simulink model "SpringMassSystemContrlledByPID"  (R2016b)
settings: Solver=ode45  StartTime=0.0  StopTime=50  MaxStep=0.05  RelTol=1e-3
libraries: simulink x1
settings Model: Creator=shyam  LastModifiedBy=shyam

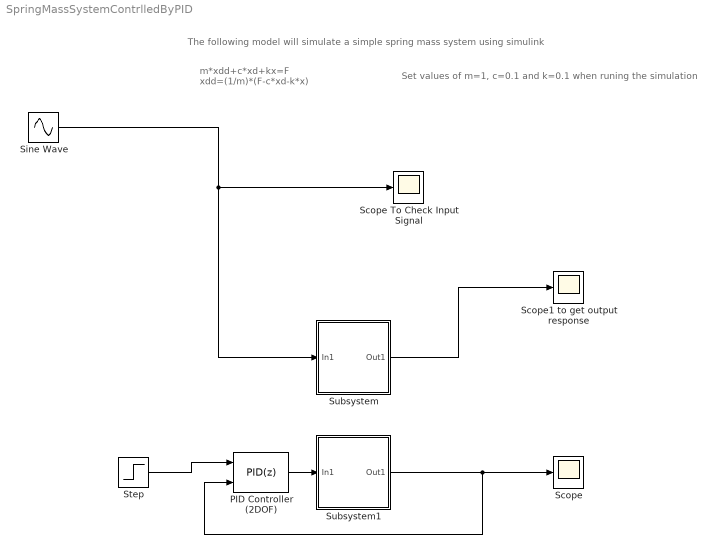
== system SpringMassSystemContrlledByPID ==
  note: Set values of m=1, c=0.1 and k=0.1 when runing the simulation
  note: The following model will simulate a simple spring mass system using simulink
  note: m*xdd+c*xd+kx=F
      | xdd=(1/m)*(F-c*xd-k*x)
  PID Controller (2DOF) : simulink/Continuous/PID Controller (2DOF)  Controller=PID  TimeDomain=Discrete-time  SampleTime=0.01  IntegratorMethod=Forward Euler  FilterMethod=Forward Euler  Form=Parallel  UseFilter=on  ControllerParametersSource=internal  P=3.93514485654865  I=0.388930047898937  D=7.6285518493241  N=88.4850232977662  b=0.926545410813894  c=0.00568917134188472  InitialConditionSource=internal  InitialConditionForIntegrator=0  InitialConditionForFilter=0  ExternalReset=none  LimitOutput=off  UpperSaturationLimit=inf  LowerSaturationLimit=-inf  LinearizeAsGain=on  AntiWindupMode=none  Kb=1  TrackingMode=off  Kt=1  PParamMin=[]  PParamMax=[]  IParamMin=[]  IParamMax=[]  DParamMin=[]  DParamMax=[]  NParamMin=[]  NParamMax=[]  bParamMin=[]  bParamMax=[]  cParamMin=[]  cParamMax=[]  KbParamMin=[]  KbParamMax=[]  KtParamMin=[]  KtParamMax=[]  POutMin=[]  POutMax=[]  IOutMin=[]  IOutMax=[]  DOutMin=[]  DOutMax=[]  NOutMin=[]  NOutMax=[]  bOutMin=[]  bOutMax=[]  cOutMin=[]  cOutMax=[]  KbOutMin=[]  KbOutMax=[]  KtOutMin=[]  KtOutMax=[]  IntegratorOutMin=[]  IntegratorOutMax=[]  FilterOutMin=[]  FilterOutMax=[]  SumOutMin=[]  SumOutMax=[]  Sum1OutMin=[]  Sum1OutMax=[]  Sum2OutMin=[]  Sum2OutMax=[]  Sum3OutMin=[]  Sum3OutMax=[]  SumI1OutMin=[]  SumI1OutMax=[]  SumI2OutMin=[]  SumI2OutMax=[]  SumI3OutMin=[]  SumI3OutMax=[]  SumDOutMin=[]  SumDOutMax=[]  SaturationOutMin=[]  SaturationOutMax=[]  IntegratorContinuousStateAttributes=''  IntegratorStateMustResolveToSignalObject=off  IntegratorRTWStateStorageClass=Auto  FilterContinuousStateAttributes=''  FilterStateMustResolveToSignalObject=off  FilterRTWStateStorageClass=Auto  DifferentiatorICPrevScaledInput=0  DifferentiatorOutMin=[]  DifferentiatorOutMax=[]
  Scope : Scope
  "Scope To Check Input Signal " : Scope
  "Scope1 to get output response " : Scope
  Sine Wave : Sin  Amplitude=2  SampleTime=0
  Step : Step  SampleTime=0
  Subsystem : Subsystem  mask{m=6, k=0.5, c=3}
      mask prompts: m "Mass"; k "Spring"; c "Damper"
  Subsystem1 : Subsystem  mask{m=6, k=0.5, c=0.1}
      mask prompts: m "Mass"; k "Spring"; c "Damper"
  wires:
  Sine Wave/1 -> Subsystem/1(In1), "Scope To Check Input Signal "/1
  Subsystem/1(Out1) -> "Scope1 to get output response "/1
  Step/1 -> PID Controller (2DOF)/1
  Subsystem1/1(Out1) -> PID Controller (2DOF)/2, Scope/1
  PID Controller (2DOF)/1 -> Subsystem1/1(In1)

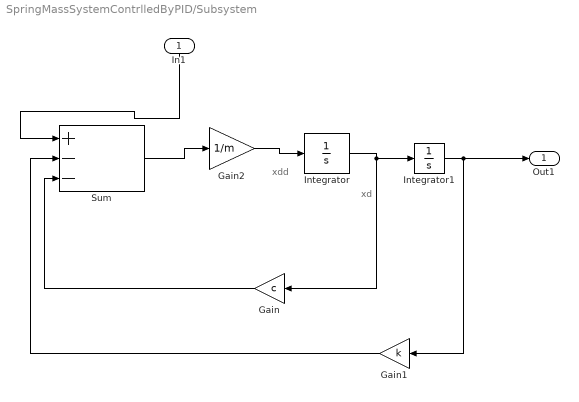
== system SpringMassSystemContrlledByPID/Subsystem ==
  note: xdd
  note: xd
  In1 : Inport
  Gain : Gain  Gain=c
  Gain1 : Gain  Gain=k
  Gain2 : Gain  Gain=1/m
  Integrator : Integrator
  Integrator1 : Integrator
  Sum : Sum  Inputs=+--
  Out1 : Outport
  wires:
  In1/1 -> Sum/1
  Sum/1 -> Gain2/1
  Integrator1/1 -> Out1/1, Gain1/1
  Integrator/1 -> Gain/1, Integrator1/1
  Gain2/1 -> Integrator/1
  Gain/1 -> Sum/3
  Gain1/1 -> Sum/2

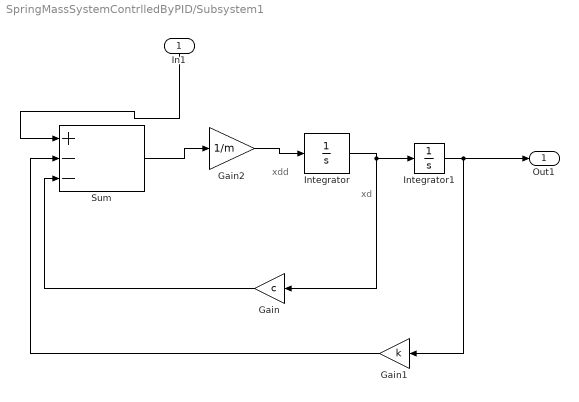
== system SpringMassSystemContrlledByPID/Subsystem1 ==
  note: xd
  note: xdd
  In1 : Inport
  Gain : Gain  Gain=c
  Gain1 : Gain  Gain=k
  Gain2 : Gain  Gain=1/m
  Integrator : Integrator
  Integrator1 : Integrator
  Sum : Sum  Inputs=+--
  Out1 : Outport
  wires:
  Gain1/1 -> Sum/2
  Gain/1 -> Sum/3
  Gain2/1 -> Integrator/1
  Integrator/1 -> Integrator1/1, Gain/1
  Integrator1/1 -> Gain1/1, Out1/1
  Sum/1 -> Gain2/1
  In1/1 -> Sum/1
